simulink model "Model_Development_backup"  (R2019a)
settings: Solver=FixedStepAuto  StartTime=0.0  StopTime=Inf  FixedStep=0.1  RelTol=1e-3
PostLoadFcn:
  | if any(exist('dsrtsu_mdlpostloadfcn', 'file') ~= 0), dsrtsu_mdlpostloadfcn('Execute', bdroot); end
InitFcn:
  | , if any(exist('rtifpga_mdlclblib', 'file') ~= 0), rtifpga_mdlclblib('Init', bdroot); end,
  | , if any(exist('dsmpb_private', 'file') ~= 0), dsmpb_private('dsmpb_mdlclblib', 'Init', bdroot); end,
libraries: dsmpblib x2
PreSaveFcn:
  | , if any(exist('dsmpb_private', 'file') ~= 0), dsmpb_private('dsmpb_mdlclblib', 'PreSave', bdroot); end,
CloseFcn:
  | , if any(exist('dsmpb_private', 'file') ~= 0), dsmpb_private('dsmpb_mdlclblib', 'Close', bdroot); end,
settings Model: DSMPB_ID_DATA={'28',struct('BlockId','9f1fea50-99ed-4d45-8ad3-952fb9fbb3f7','SignalIds',{{'3f5e9160-ecb2-4fe5-bf14-617dbef05cb2'}}),'31',struct('BlockId','10894696-7aac-4333-a05e-37f13e0eedfc','SignalIds',{{'d61dd94f-0b03-43b6-9401-8b62f8eb8c9e','703cc474-4f8c-426e-980c-7f3b47c6f237','283ba769-de60-4e66-8dae-9c9288764590','6a7dd420-ff6f-4b9d-b626-112f75dcf41e','74e8e34e-38ec-4726-b97a-e21645c081c3'}})}  RTICANMMDATA=struct('GeneralSetupData',struct('modelroot','C:\Users\RCP-Lab\Documents\00_Projekte\00_MODEL\Development_Ajay','generalsettings',struct('filesettings',struct('destfolder',struct('Name','RTICANMM_FILES','Check',1),'buildfolder',struct('Name','.','Check',1),'AbsDestfolder',struct('Name','C:\Users\RCP-Lab\Documents\00_Projekte\00_MODEL\Development_Ajay\RTICANMM_FILES'),'AbsBuildfolder',struct('Name','C:\Users\RCP-Lab\Documents\00_Projekte\00_MODEL\Development_Ajay'))),'options',struct('addpaths',1,'rmpaths',1,'addtrcexclusion',true,'cannavigator',struct('checkmonitoring',0),'show_usrtrc',0,'use_usrtrc',0),'advanced',struct('options',ones(1,100)),'MPSetup',{{}},'RTI',struct('Type','DSRT','Ver','4.3','Date','02-May-2020'),'modelname','Model_Development','block','Model_Development'))  DSRTSU_INTERNAL_RTIFPGA=160  Creator=RCP-Lab  LastModifiedBy=RCP-Lab
settings OptimizationCC: BlockReduction=off  ConditionallyExecuteInputs=off  OptimizeBlockIOStorage=off  BufferReuse=off  GlobalBufferReuse=off  ExpressionFolding=off  LocalBlockOutputs=off  OptimizeDataStoreBuffers=off  BusAssignmentInplaceUpdate=off
settings DebuggingCC: TasksWithSamePriorityMsg=none
settings HardwareCC: ProdBitPerPointer=32  ProdBitPerSizeT=32  ProdBitPerPtrDiffT=32  ProdLargestAtomicInteger=Integer  ProdWordSize=32  ProdLongLongMode=on  ProdHWDeviceType=Custom Processor->Custom
settings ModelReferenceCC: EnableParallelModelReferenceBuilds=on
settings SFSimCC: MATLABDynamicMemAlloc=off
settings RTWCC: SystemTargetFile=dsrt.tlc  GenCodeOnly=on  MakeCommand=make_dsrt  TemplateMakefile=dsrt_default_tmf  Description=dSPACE Run-Time Target (for VEOS on Windows and ConfigurationDesk)  RTWVerbose=off
settings STFCustomTargetCC: TargetLangStandard=C99 (ISO)  ParMdlRefBuildCompliant=on  GRTInterface=off  SystemTargetFile=dsrt.tlc
settings GRTTargetCC: CompOptLevelCompliant=off  ConcurrentExecutionCompliant=off  CombineOutputUpdateFcns=off  MatFileLogging=off  CPPClassGenCompliant=off  UseToolchainInfoCompliant=off

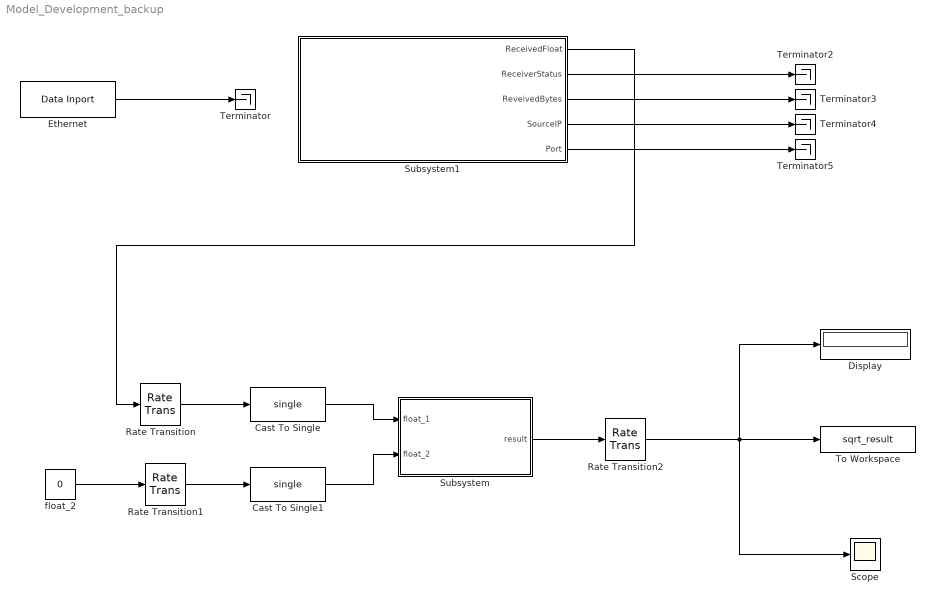
== system Model_Development_backup ==
  Cast To Single : DataTypeConversion  OutDataTypeStr=single
  Cast To Single1 : DataTypeConversion  OutDataTypeStr=single
  Display : Display
  Ethernet : dsmpblib/Data Inport  Priority=10000
      settings: SourceProductName=dSPACE Model Interface Blockset
  Rate Transition : RateTransition
  Rate Transition1 : RateTransition
  Rate Transition2 : RateTransition  OutPortSampleTime=5
  Scope : Scope
  Subsystem : Subsystem
  Subsystem1 : Subsystem
  Terminator{,2..5} (5 alike) : Terminator
  To Workspace : ToWorkspace  VariableName=sqrt_result  SaveFormat=Timeseries  SampleTime=-1
  float_2 : Constant  Value=0
  wires:
  Subsystem/1(result) -> Rate Transition2/1
  Cast To Single/1 -> Subsystem/1(float_1)
  Cast To Single1/1 -> Subsystem/2(float_2)
  float_2/1 -> Rate Transition1/1
  Rate Transition/1 -> Cast To Single/1
  Rate Transition1/1 -> Cast To Single1/1
  Rate Transition2/1 -> Scope/1, To Workspace/1, Display/1
  Ethernet/1 -> Terminator/1
  Subsystem1/2(ReceiverStatus) -> Terminator2/1
  Subsystem1/3(ReveivedBytes) -> Terminator3/1
  Subsystem1/4(SourceIP) -> Terminator4/1
  Subsystem1/5(Port) -> Terminator5/1
  Subsystem1/1(ReceivedFloat) -> Rate Transition/1

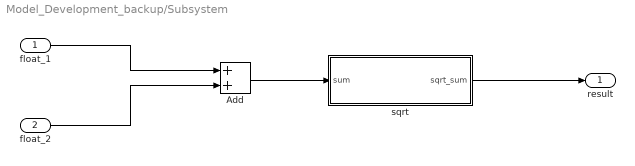
== system Model_Development_backup/Subsystem ==
  float_1 : Inport
  float_2 : Inport  Port=2
  Add : Sum
  sqrt : MATLAB Function  TreatAsAtomicUnit=on
  result : Outport
  wires:
  Add/1 -> sqrt/1(sum)
  float_1/1 -> Add/1
  float_2/1 -> Add/2
  sqrt/1(sqrt_sum) -> result/1

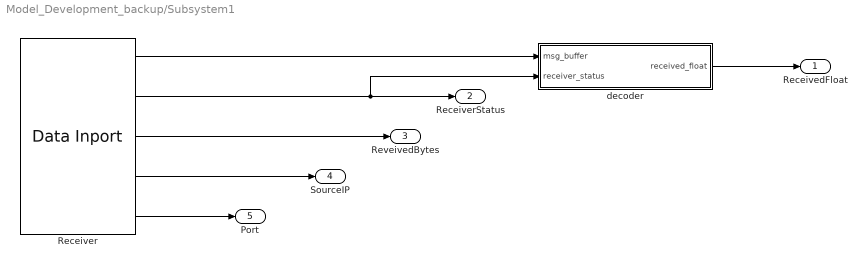
== system Model_Development_backup/Subsystem1 ==
  Receiver : dsmpblib/Data Inport  Priority=10000
      settings: SourceProductName=dSPACE Model Interface Blockset
  decoder : MATLAB Function  TreatAsAtomicUnit=on
  ReceivedFloat : Outport
  ReceiverStatus : Outport  Port=2
  ReveivedBytes : Outport  Port=3
  SourceIP : Outport  Port=4
  Port : Outport  Port=5
  wires:
  Receiver/3 -> ReveivedBytes/1
  Receiver/4 -> SourceIP/1
  Receiver/2 -> decoder/2(receiver_status), ReceiverStatus/1
  Receiver/5 -> Port/1
  Receiver/1 -> decoder/1(msg_buffer)
  decoder/1(received_float) -> ReceivedFloat/1

== matlab function Model_Development_backup/Subsystem1/decoder ==
  data: msg_buffer input; received_float output; receiver_status input
function received_float = fcn(msg_buffer, receiver_status)

received_float = single(0);

if isempty(msg_buffer) || ~receiver_status
    return;
else
    %shape_bytes = read(msg_buffer, 8);
    %data = typecast(uint8(shape_bytes), 'uint32');
    received_float = typecast(msg_buffer, 'single');
end

end

== matlab function Model_Development_backup/Subsystem/sqrt ==
  data: sum input; sqrt_sum output
function sqrt_sum = fcn(sum)

sqrt_sum = sum

%sqrt_sum = square_root(sum);

end
